simulink model "p5p5d_sim"  (Simulink 8.9)
settings: Solver=ode45  StartTime=0.0  StopTime=500  RelTol=1e-3  EnableMultiTasking=on
values from neighbouring files (symbols this model uses):
  K_pd = 0.841    [p5p5c.m]    (also in p5p5d.m = 0.839; p5p5e.m)
  T_d = T    [p5p5c.m]    (also in p5p5d.m; p5p5e.m)
  T_f = 8.35    [p5p5c.m]    (also in p5p5d.m = 8.4; p5p5e.m)
  T_s = 0.1    [p5p5c.m]    (also in p5p5d.m; p5p5e.m)
libraries: simulink x2
settings Model: Creator=markh  LastModifiedBy=thobern
settings DataIOCC: SignalLoggingName=sigsOut
settings OptimizationCC: InitFltsAndDblsToZero=on
settings DebuggingCC: SaveWithParameterizedLinksMsg=none  SignalResolutionControl=TryResolveAllWithWarning  MultiTaskDSMMsg=warning  MultiTaskCondExecSysMsg=none
settings HardwareCC: TargetUnknown=on
settings GRTTargetCC: TargetFcnLib=ansi_tfl_tmw.mat

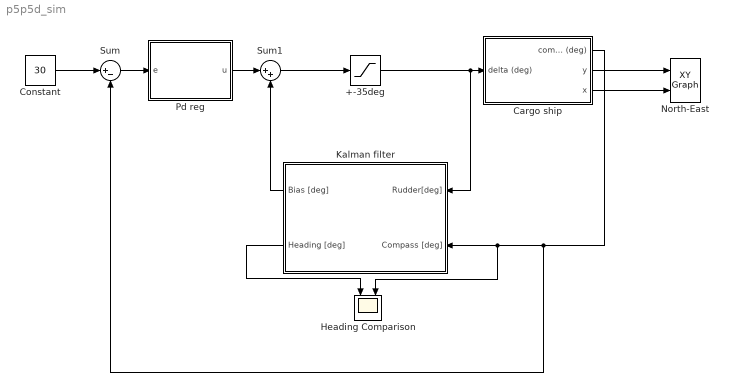
== system p5p5d_sim ==
  +-35deg : Saturate  UpperLimit=35  LowerLimit=-35
  Cargo ship : Subsystem  mask(Simple shipmodel for a cargo ship){noise=on, current=on, logic=off}
      mask prompts: noise "measurement noise"; logic "waves"
      mask help:
      | Measurement noise:
      | 	checked = noise on
      | 	unchecked = noise off
      |
      | Current:
      | 	checked = current on
      | 	unchecked = current off
      |
      | Waves:
      | 	checked = waves on
      | 	unchecked = waves off
      |
      | Author: Jørgen Spjøtvold, 9/10-2003
      | TTK 4115 Linear system theory.
      | Modified by Jostein Bakkeheim 26/10-2006
  Constant : Constant  Value=30
  Heading Comparison : Scope  NumInputPorts=2
  Kalman filter : Subsystem
  North-East : simulink/Sinks/XY Graph  xmin=-5000  xmax=5000  ymin=-5000  ymax=5000  st=-1
  "Pd reg " : Subsystem
  Sum : Sum  Inputs=|+-
  Sum1 : Sum  Inputs=|++
  wires:
  Cargo ship/3(x) -> North-East/2
  Cargo ship/2(y) -> North-East/1
  Sum/1 -> "Pd reg "/1(e)
  Constant/1 -> Sum/1
  "Pd reg "/1("u ") -> Sum1/1
  Cargo ship/1(compass (deg)) -> Sum/2, Kalman filter/2(Compass [deg]), Heading Comparison/2
  Sum1/1 -> +-35deg/1
  +-35deg/1 -> Kalman filter/1(Rudder[deg]), Cargo ship/1(delta (deg))
  Kalman filter/2(Heading [deg]) -> Heading Comparison/1
  Kalman filter/1(Bias [deg]) -> Sum1/2

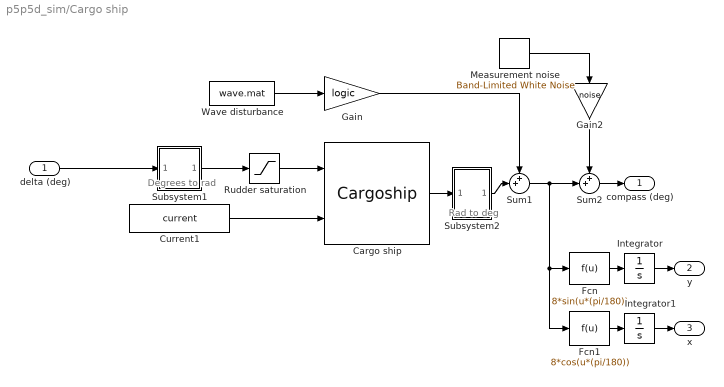
== system p5p5d_sim/Cargo ship ==
  note: Degrees to rad
  note: Rad to deg
  delta (deg) : Inport
  Cargo ship : S-Function  FunctionName=Cargoship  SFunctionDeploymentMode=off  EnableBusSupport=off  mask(Cargo ship){}
      mask help:
      | S-function which simulates a cargo ship.
      |
      | Author: Jørgen Spjøtvold
      | 20.10-2003
      | Modified by Jostein Bakkeheim 27.10.2006
  Current1 : Constant  Value=current
  Fcn : Fcn  Expr=8*sin(u*(pi/180))
  Fcn1 : Fcn  Expr=8*cos(u*(pi/180))
  Gain : Gain  Gain=logic  SaturateOnIntegerOverflow=on  OutDataTypeStr=Inherit: Same as input  ParamDataTypeStr=Inherit: Same as input
  Gain2 : Gain  Gain=noise  SaturateOnIntegerOverflow=on  OutDataTypeStr=Inherit: Same as input  ParamDataTypeStr=Inherit: Same as input
  Integrator : Integrator
  Integrator1 : Integrator
  Measurement noise : simulink/Sources/Band-Limited White Noise  Cov=[0.001]  Ts=.5  seed=[23341]
  Rudder saturation : Saturate  UpperLimit=45*(pi/180)  LowerLimit=-45*(pi/180)
  Subsystem1 : Subsystem  mask(degrees to radians){}
      mask help: Converts degrees to radians
      mask Display: fprintf('D2R');
  Subsystem2 : Subsystem  mask(radians to degrees){}
      mask help: Converts radians to degrees
      mask Display: fprintf('R2D');
  Sum1 : Sum  Inputs=++|  SaturateOnIntegerOverflow=on
  Sum2 : Sum  Inputs=++|  SaturateOnIntegerOverflow=on
  Wave disturbance : FromFile  FileName=wave.mat  SampleTime=0
  compass (deg) : Outport
  y : Outport  Port=2
  x : Outport  Port=3
  wires:
  delta (deg)/1 -> Subsystem1/1(In1)
  Fcn/1 -> Integrator/1
  Integrator/1 -> y/1
  Fcn1/1 -> Integrator1/1
  Integrator1/1 -> x/1
  Wave disturbance/1 -> Gain/1
  Subsystem2/1(Out1) -> Sum1/2
  Gain/1 -> Sum1/1
  Sum1/1 -> Fcn/1, Fcn1/1, Sum2/2
  Cargo ship/1 -> Subsystem2/1(In1)
  Subsystem1/1(Out1) -> Rudder saturation/1
  Rudder saturation/1 -> Cargo ship/1
  Sum2/1 -> compass (deg)/1
  Measurement noise/1 -> Gain2/1
  Gain2/1 -> Sum2/1
  Current1/1 -> Cargo ship/2

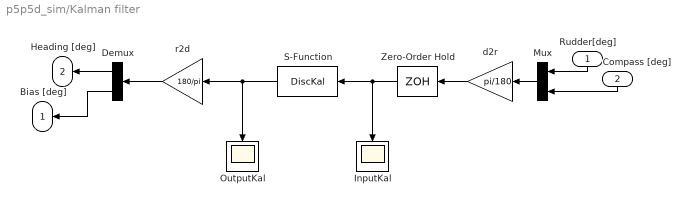
== system p5p5d_sim/Kalman filter ==
  Rudder[deg] : Inport
  Compass [deg] : Inport  Port=2
  Demux : Demux  Outputs=2
  InputKal : Scope
  Mux : Mux  Inputs=2
  OutputKal : Scope
  S-Function : S-Function  FunctionName=DiscKal  Parameters=data  SFunctionModules='DiscKal'  SFunctionDeploymentMode=off  EnableBusSupport=off
  Zero-Order Hold : ZeroOrderHold  SampleTime=T_s
  d2r : Gain  Gain=pi/180
  r2d : Gain  Gain=180/pi
  Bias [deg] : Outport
  Heading [deg] : Outport  Port=2
  wires:
  d2r/1 -> Zero-Order Hold/1
  Demux/1 -> Heading [deg]/1
  Zero-Order Hold/1 -> S-Function/1, InputKal/1
  S-Function/1 -> r2d/1, OutputKal/1
  Mux/1 -> d2r/1
  Demux/2 -> Bias [deg]/1
  Rudder[deg]/1 -> Mux/1
  Compass [deg]/1 -> Mux/2
  r2d/1 -> Demux/1

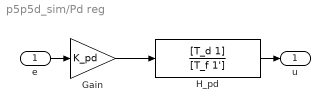
== system p5p5d_sim/Pd reg  ==
  e : Inport
  Gain : Gain  Gain=K_pd
  H_pd : TransferFcn  Numerator=[T_d 1]  Denominator=[T_f 1']
  "u " : Outport
  wires:
  Gain/1 -> H_pd/1
  H_pd/1 -> "u "/1
  e/1 -> Gain/1

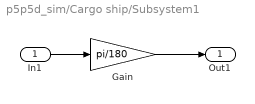
== system p5p5d_sim/Cargo ship/Subsystem1 ==
  In1 : Inport
  Gain : Gain  Gain=pi/180  SaturateOnIntegerOverflow=on  OutDataTypeStr=Inherit: Same as input  ParamDataTypeStr=Inherit: Same as input
  Out1 : Outport
  wires:
  Gain/1 -> Out1/1
  In1/1 -> Gain/1

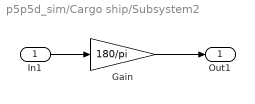
== system p5p5d_sim/Cargo ship/Subsystem2 ==
  In1 : Inport
  Gain : Gain  Gain=180/pi  SaturateOnIntegerOverflow=on  OutDataTypeStr=Inherit: Same as input  ParamDataTypeStr=Inherit: Same as input
  Out1 : Outport
  wires:
  Gain/1 -> Out1/1
  In1/1 -> Gain/1
